simulink model "observer_sim"  (R2020a)
settings: Solver=VariableStepAuto  StartTime=0.0  StopTime=5  RelTol=1e-6
undefined symbols (not defined in the file): A, B, C, C_full, D_full, icd, K, L
settings Model: Creator=Jasper  LastModifiedBy=Jasper

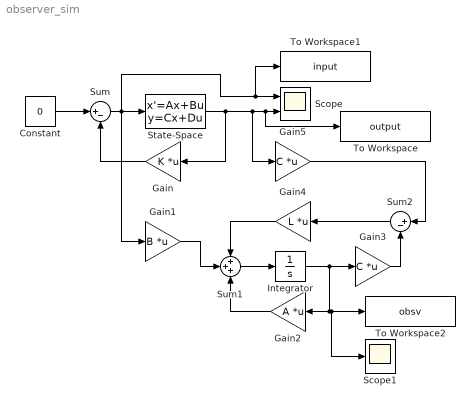
== system observer_sim ==
  Constant : Constant  Value=0
  Gain : Gain  Gain=K  Multiplication=Matrix(K*u)
  Gain1 : Gain  Gain=B  Multiplication=Matrix(K*u)
  Gain2 : Gain  Gain=A  Multiplication=Matrix(K*u)
  Gain3 : Gain  Gain=C  Multiplication=Matrix(K*u)
  Gain4 : Gain  Gain=L  Multiplication=Matrix(K*u)
  Gain5 : Gain  Gain=C  Multiplication=Matrix(K*u)
  Integrator : Integrator  InitialCondition=[0.1 0.1 0 0]
  Scope : Scope  NumInputPorts=2
  Scope1 : Scope
  State-Space : StateSpace  A=A  B=B  C=C_full  D=D_full  InitialCondition=icd
  Sum : Sum  Inputs=|+-
  Sum1 : Sum  Inputs=+++
  Sum2 : Sum  Inputs=|+-
  To Workspace : ToWorkspace  VariableName=output  SaveFormat=Timeseries  SampleTime=-1
  To Workspace1 : ToWorkspace  VariableName=input  SaveFormat=Timeseries  SampleTime=-1
  To Workspace2 : ToWorkspace  VariableName=obsv  SaveFormat=Timeseries  SampleTime=-1
  wires:
  State-Space/1 -> Gain5/1, To Workspace/1, Scope/2, Gain/1
  Gain/1 -> Sum/2
  Sum/1 -> Gain1/1, To Workspace1/1, Scope/1, State-Space/1
  Constant/1 -> Sum/1
  Sum1/1 -> Integrator/1
  Integrator/1 -> Gain3/1, Gain2/1, Scope1/1, To Workspace2/1
  Gain3/1 -> Sum2/2
  Gain1/1 -> Sum1/2
  Gain2/1 -> Sum1/3
  Sum2/1 -> Gain4/1
  Gain4/1 -> Sum1/1
  Gain5/1 -> Sum2/1
